simulink model "MPC_Observer"  (R2015a)
settings: Solver=ode14x  StartTime=0.0  StopTime=Total_t_sim  FixedStep=dt  RelTol=1e-3
values from neighbouring files (symbols this model uses):
  A = F    [DMPC_AVC.m]    (also in DMPC_AVC_imp.m)
  A_cons = [L_m;-L_m]    [DMPC_AVC.m]    (also in DMPC_AVC_imp.m)
  A_nom = A    [DMPC_AVC.m]
  B = G    [DMPC_AVC.m]    (also in DMPC_AVC_imp.m)
  B_nom = B    [DMPC_AVC.m]
  C = H    [DMPC_AVC.m]    (also in DMPC_AVC_imp.m)
  C_nom = C    [DMPC_AVC.m]
  coefs = coefs(1,2:end)    [DMPC_AVC.m]    (also in DMPC_AVC_imp.m)
  dt = 2e-4    (= 0.0002)    [DMPC_AVC.m]    (also in DMPC_AVC_imp.m = 0.001)
  H_nom = H    [DMPC_AVC.m]
  L2 = dlqr(A',C',1e-11*eye(size(A)),1e-7)'    [DMPC_AVC.m]
  u_bound = [u_max;-u_min]    [DMPC_AVC.m]    (also in DMPC_AVC_imp.m)
undefined symbols (not defined in the file or in its folder): L_m, omega, psi
settings Model: Creator=Ablah  LastModifiedBy=Ablah

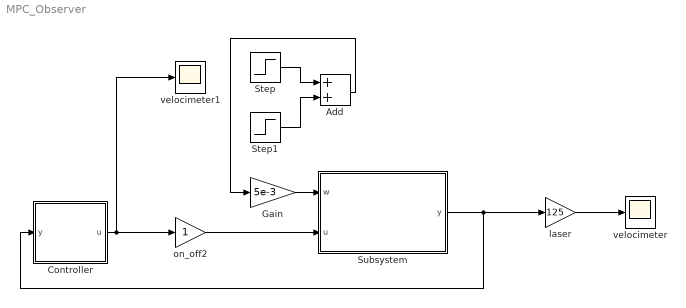
== system MPC_Observer ==
  Add : Sum
  Controller : Subsystem
  Gain : Gain  Gain=5e-3
  Step : Step  SampleTime=0
  Step1 : Step  Time=1.01  After=-1  SampleTime=0
  Subsystem : Subsystem
  laser : Gain  Gain=125
  on_off2 : Gain
  velocimeter : Scope
      settings: YMin=-10  YMax=10
  velocimeter1 : Scope
      settings: YMin=-2.25  YMax=2.25  SaveName=ScopeData5
  wires:
  Add/1 -> Gain/1
  Controller/1(u) -> velocimeter1/1, on_off2/1
  laser/1 -> velocimeter/1
  Gain/1 -> Subsystem/1(w)
  Subsystem/1(y) -> Controller/1(y), laser/1
  on_off2/1 -> Subsystem/2(u)
  Step/1 -> Add/1
  Step1/1 -> Add/2

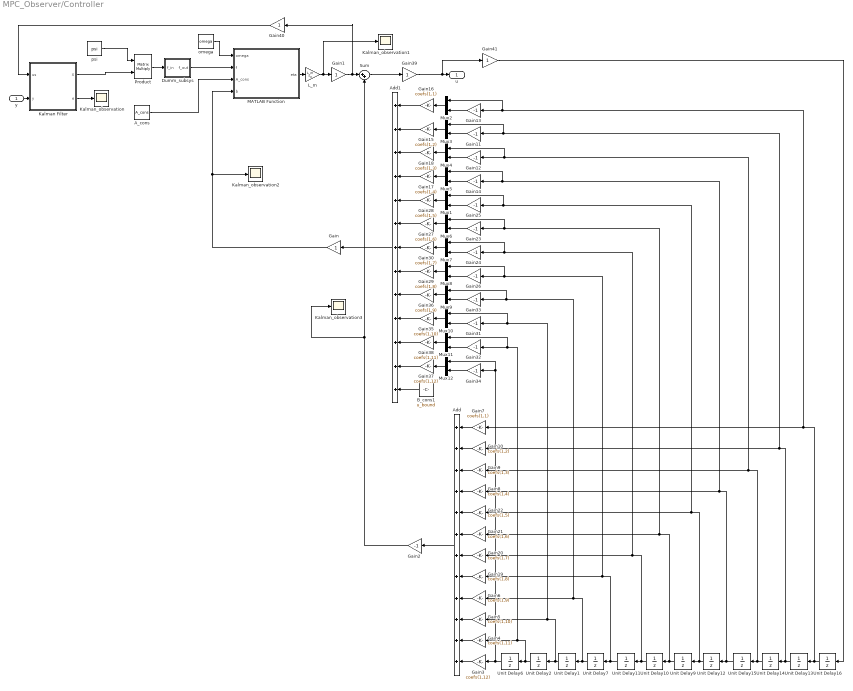
== system MPC_Observer/Controller ==
  y : Inport
  A_cons : Constant  Value=A_cons  SampleTime=dt
  Add : Sum  Inputs=++++++++++++
  Add1 : Sum  Inputs=+++++++++++++
  B_cons1 : Constant  Value=u_bound
  Dumm_subsys : Subsystem
  Gain{,1,39..41} (5 alike) : Gain
  Gain10 : Gain  Gain=coefs(1,2)
  Gain{2,11..14,23..26,31..34} (13 alike) : Gain  Gain=-1
  Gain15 : Gain  Gain=coefs(1,2)
  Gain16 : Gain  Gain=coefs(1,1)
  Gain17 : Gain  Gain=coefs(1,4)
  Gain18 : Gain  Gain=coefs(1,3)
  Gain19 : Gain  Gain=coefs(1,8)
  Gain20 : Gain  Gain=coefs(1,7)
  Gain21 : Gain  Gain=coefs(1,6)
  Gain22 : Gain  Gain=coefs(1,5)
  Gain27 : Gain  Gain=coefs(1,6)
  Gain28 : Gain  Gain=coefs(1,5)
  Gain29 : Gain  Gain=coefs(1,8)
  Gain3 : Gain  Gain=coefs(1,12)
  Gain30 : Gain  Gain=coefs(1,7)
  Gain35 : Gain  Gain=coefs(1,10)
  Gain36 : Gain  Gain=coefs(1,9)
  Gain37 : Gain  Gain=coefs(1,12)
  Gain38 : Gain  Gain=coefs(1,11)
  Gain4 : Gain  Gain=coefs(1,11)
  Gain5 : Gain  Gain=coefs(1,10)
  Gain6 : Gain  Gain=coefs(1,9)
  Gain7 : Gain  Gain=coefs(1,1)
  Gain8 : Gain  Gain=coefs(1,4)
  Gain9 : Gain  Gain=coefs(1,3)
  Kalman Filter : Subsystem  TreatAsAtomicUnit=on
      settings: MinAlgLoopOccurrences=on
  Kalman_observation{,1..3} (4 alike) : Scope
      Kalman_observation settings: YMin=-3.5e-11  YMax=3.5e-11
      Kalman_observation1 settings: YMin=-0.000155  YMax=-6.5e-05  SaveName=ScopeData2
      Kalman_observation2 settings: YMin=-0.000155  YMax=-6.5e-05  SaveName=ScopeData6
      Kalman_observation3 settings: YMin=-0.000155  YMax=-6.5e-05  SaveName=ScopeData4
  L_m : Gain  Gain=L_m  Multiplication=Matrix(K*u)
  MATLAB Function : MATLAB Function  TreatAsAtomicUnit=on
      settings: MinAlgLoopOccurrences=on
  Mux{1..12} (12 alike) : Mux  Inputs=2
  Product : Product  Multiplication=Matrix(*)  RndMeth=Zero
  Sum : Sum  Inputs=|++
  Unit Delay{1..2,6..7,9..16} (12 alike) : UnitDelay  SampleTime=dt
  omega : Constant  Value=omega  SampleTime=dt
  psi : Constant  Value=psi  SampleTime=dt
  u : Outport
  wires:
  MATLAB Function/1(eta) -> L_m/1
  L_m/1 -> Kalman_observation1/1, Gain1/1
  omega/1 -> MATLAB Function/1(omega)
  A_cons/1 -> MATLAB Function/3(A_cons)
  psi/1 -> Product/1
  y/1 -> Kalman Filter/2(y)
  Gain7/1 -> Add/1
  Gain9/1 -> Add/3
  Gain8/1 -> Add/4
  Gain13/1 -> Mux2/2
  Gain11/1 -> Mux3/2
  Gain12/1 -> Mux4/2
  Gain14/1 -> Mux5/2
  Mux2/1 -> Gain16/1
  Mux3/1 -> Gain15/1
  Mux4/1 -> Gain18/1
  Mux5/1 -> Gain17/1
  Gain16/1 -> Add1/1
  Gain15/1 -> Add1/2
  Gain18/1 -> Add1/3
  Gain17/1 -> Add1/4
  Add/1 -> Gain2/1
  Gain10/1 -> Add/2
  Product/1 -> Dumm_subsys/1(f_in)
  Dumm_subsys/1(f_out) -> MATLAB Function/2(f)
  Kalman Filter/1(X) -> Product/2
  Kalman Filter/2(e) -> Kalman_observation/1
  Gain1/1 -> Sum/1, Gain40/1
  Unit Delay2/1 -> Mux11/1, Gain32/1, Gain4/1, Unit Delay6/1
  Unit Delay1/1 -> Mux10/1, Gain31/1, Gain5/1, Unit Delay2/1
  Unit Delay7/1 -> Gain6/1, Mux9/1, Gain33/1, Unit Delay1/1
  Unit Delay11/1 -> Mux8/1, Gain26/1, Gain19/1, Unit Delay7/1
  Unit Delay10/1 -> Mux7/1, Gain24/1, Gain20/1, Unit Delay11/1
  Unit Delay9/1 -> Mux6/1, Gain23/1, Gain21/1, Unit Delay10/1
  Unit Delay12/1 -> Mux1/1, Gain25/1, Gain22/1, Unit Delay9/1
  Unit Delay15/1 -> Gain14/1, Mux5/1, Gain8/1, Unit Delay12/1
  Unit Delay14/1 -> Mux4/1, Gain12/1, Gain9/1, Unit Delay15/1
  Unit Delay13/1 -> Mux3/1, Gain11/1, Gain10/1, Unit Delay14/1
  Unit Delay16/1 -> Mux2/1, Gain13/1, Gain7/1, Unit Delay13/1
  Gain3/1 -> Add/12
  Unit Delay6/1 -> Gain34/1, Mux12/1, Gain3/1
  Gain4/1 -> Add/11
  Gain5/1 -> Add/10
  Gain6/1 -> Add/9
  Gain19/1 -> Add/8
  Gain20/1 -> Add/7
  Gain21/1 -> Add/6
  Gain22/1 -> Add/5
  B_cons1/1 -> Add1/13
  Gain25/1 -> Mux1/2
  Gain23/1 -> Mux6/2
  Gain24/1 -> Mux7/2
  Gain26/1 -> Mux8/2
  Mux1/1 -> Gain28/1
  Mux6/1 -> Gain27/1
  Mux7/1 -> Gain30/1
  Mux8/1 -> Gain29/1
  Gain33/1 -> Mux9/2
  Gain31/1 -> Mux10/2
  Gain32/1 -> Mux11/2
  Gain34/1 -> Mux12/2
  Mux9/1 -> Gain36/1
  Mux10/1 -> Gain35/1
  Mux11/1 -> Gain38/1
  Mux12/1 -> Gain37/1
  Gain28/1 -> Add1/5
  Gain27/1 -> Add1/6
  Gain30/1 -> Add1/7
  Gain29/1 -> Add1/8
  Gain36/1 -> Add1/9
  Gain35/1 -> Add1/10
  Gain38/1 -> Add1/11
  Gain37/1 -> Add1/12
  Sum/1 -> Gain39/1
  Gain2/1 -> Kalman_observation3/1, Sum/2
  Gain39/1 -> Gain41/1, u/1
  Gain40/1 -> Kalman Filter/1(us)
  Gain41/1 -> Unit Delay16/1
  Add1/1 -> Gain/1
  Gain/1 -> Kalman_observation2/1, MATLAB Function/4(b)

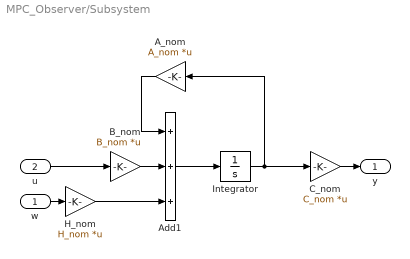
== system MPC_Observer/Subsystem ==
  w : Inport
  u : Inport  Port=2
  A_nom : Gain  Gain=A_nom  Multiplication=Matrix(K*u)
  Add1 : Sum  Inputs=+++
  B_nom : Gain  Gain=B_nom  Multiplication=Matrix(K*u)
  "C_nom " : Gain  Gain=C_nom  Multiplication=Matrix(K*u)
  H_nom : Gain  Gain=H_nom  Multiplication=Matrix(K*u)
  Integrator : Integrator
  y : Outport
  wires:
  "C_nom "/1 -> y/1
  Add1/1 -> Integrator/1
  A_nom/1 -> Add1/1
  H_nom/1 -> Add1/3
  Integrator/1 -> "C_nom "/1, A_nom/1
  B_nom/1 -> Add1/2
  u/1 -> B_nom/1
  w/1 -> H_nom/1

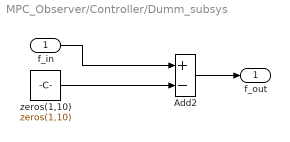
== system MPC_Observer/Controller/Dumm_subsys ==
  f_in : Inport
  Add2 : Sum  Inputs=+-
  zeros(1,10) : Constant  Value=zeros(1,10)  SampleTime=dt
  f_out : Outport
  wires:
  f_in/1 -> Add2/1
  Add2/1 -> f_out/1
  zeros(1,10)/1 -> Add2/2

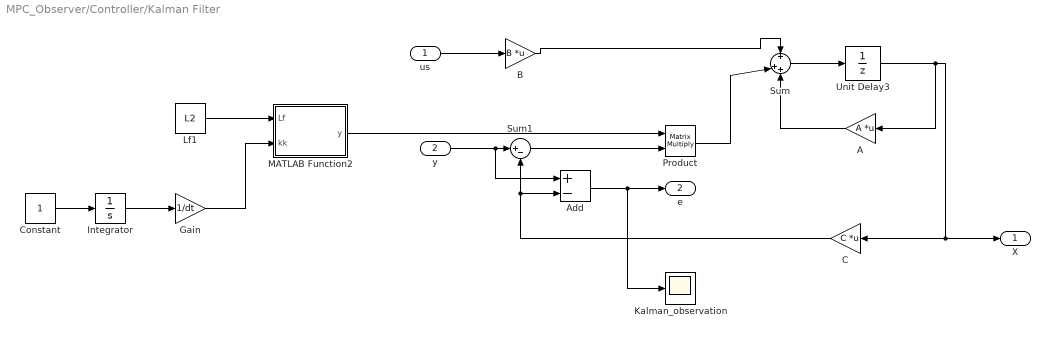
== system MPC_Observer/Controller/Kalman Filter ==
  us : Inport
  y : Inport  Port=2
  A : Gain  Gain=A  Multiplication=Matrix(K*u)
  Add : Sum  Inputs=+-
  B : Gain  Gain=B  Multiplication=Matrix(K*u)
  C : Gain  Gain=C  Multiplication=Matrix(K*u)
  Constant : Constant
  Gain : Gain  Gain=1/dt
  Integrator : Integrator
  Kalman_observation : Scope
      settings: YMin=-8e-13  YMax=7e-13  SaveName=ScopeData3
  Lf1 : Constant  Value=L2
  MATLAB Function2 : MATLAB Function  TreatAsAtomicUnit=on
      settings: MinAlgLoopOccurrences=on
  Product : Product  Multiplication=Matrix(*)  RndMeth=Zero
  Sum : Sum  Inputs=+|++
  Sum1 : Sum  Inputs=|+-
  Unit Delay3 : UnitDelay  SampleTime=dt
  X : Outport
  e : Outport  Port=2
  wires:
  Unit Delay3/1 -> A/1, X/1, C/1
  A/1 -> Sum/3
  Sum/1 -> Unit Delay3/1
  us/1 -> B/1
  B/1 -> Sum/1
  C/1 -> Add/2, Sum1/2
  y/1 -> Add/1, Sum1/1
  Sum1/1 -> Product/2
  Product/1 -> Sum/2
  Lf1/1 -> MATLAB Function2/1(Lf)
  MATLAB Function2/1(y) -> Product/1
  Constant/1 -> Integrator/1
  Integrator/1 -> Gain/1
  Gain/1 -> MATLAB Function2/2(kk)
  Add/1 -> Kalman_observation/1, e/1

== matlab function MPC_Observer/Controller/MATLAB Function ==
  data: omega input; eta output; f input; A_cons input; b input
function eta=QPomegaild(omega,f,A_cons,b)

[n1,m1]=size(A_cons);
% eta=-omega\f;
eta=-inv(omega)*f;
kk=0;
for i=1:n1
    if (A_cons(i,:)*eta>b(i)) 
        kk=kk+1;
    else
        kk=kk+0;
    end
end
if (kk==0)
    return
end
P=A_cons*(omega\A_cons');
d=(A_cons*(omega\f)+b);
[n,m]=size(d);
x_ini=zeros(n,m);
lambda=x_ini;
% al=10;
for km=1:38

%find tomegae elements in tomegae solution vector one by one
% km could be larger if tomegae Lagranger multiplier omegaas a slow
% convergence rate.
    lambda_p=lambda;
    for i=1:n
        w= P(i,:)*lambda-P(i,i)*lambda(i,1);
        w=w+d(i,1);
        la=-w/P(i,i);
        lambda(i,1)=max(0,la);
    end
    
    al=(lambda-lambda_p)'*(lambda-lambda_p);
    if (al<10e-30)
        break;
    end
 end
eta=-omega\f -omega\A_cons'*lambda;

== matlab function MPC_Observer/Controller/Kalman Filter/MATLAB Function2 ==
  data: y output; Lf input; kk input
function y = fcn(Lf,kk)
%#eml

% kk1 = floor(kk)+1;
% 
% y = Lf(:,kk1);
y = Lf;
